simulink model "ECGdenoising_systemgenerator"  (R2018a)
settings: Solver=VariableStepAuto  StartTime=0.0  StopTime=10800  RelTol=1e-3
libraries: xbsIndex_r4 x811, dspsrcs4 x1
(part 3 of 3)

== system ECGdenoising_systemgenerator/DWT block Reference Signal generation/Low Pass Reconstruction 4 ==
  In3 : Inport
  AddSub{14..20} (7 alike) : xbsIndex_r4/AddSub  mode=Addition  use_carryin=off  use_carryout=off  en=off  latency=0  precision=User Defined  arith_type="Signed  (2's comp)"  n_bits=16  bin_pt=14  quantization=Truncate  overflow=Saturate  use_behavioral_HDL=off  hw_selection=Fabric  pipelined=off  dbl_ovrd=off  block_type=addsub
  Constant16 : xbsIndex_r4/Constant  const=0.6308807679  gui_display_data_type=Fixed-point  arith_type=Signed (2's comp)  n_bits=16  bin_pt=14  preci_type=Single  exp_width=8  frac_width=24  explicit_period=on  period=64  equ=P=C  opselect=C  inp2=PCIN>>17  opr=+  inp1=P  carry=CIN  dbl_ovrd=off  block_type=constant
  Constant17 : xbsIndex_r4/Constant  const=-0.0279837694  gui_display_data_type=Fixed-point  arith_type=Signed (2's comp)  n_bits=16  bin_pt=14  preci_type=Single  exp_width=8  frac_width=24  explicit_period=on  period=64  equ=P=C  opselect=C  inp2=PCIN>>17  opr=+  inp1=P  carry=CIN  dbl_ovrd=off  block_type=constant
  Constant18 : xbsIndex_r4/Constant  const=-0.1870348117  gui_display_data_type=Fixed-point  arith_type=Signed (2's comp)  n_bits=16  bin_pt=14  preci_type=Single  exp_width=8  frac_width=24  explicit_period=on  period=64  equ=P=C  opselect=C  inp2=PCIN>>17  opr=+  inp1=P  carry=CIN  dbl_ovrd=off  block_type=constant
  Constant19 : xbsIndex_r4/Constant  const=0.0308413818  gui_display_data_type=Fixed-point  arith_type=Signed (2's comp)  n_bits=16  bin_pt=14  preci_type=Single  exp_width=8  frac_width=24  explicit_period=on  period=64  equ=P=C  opselect=C  inp2=PCIN>>17  opr=+  inp1=P  carry=CIN  dbl_ovrd=off  block_type=constant
  Constant20 : xbsIndex_r4/Constant  const=0.0328830117  gui_display_data_type=Fixed-point  arith_type=Signed (2's comp)  n_bits=16  bin_pt=14  preci_type=Single  exp_width=8  frac_width=24  explicit_period=on  period=64  equ=P=C  opselect=C  inp2=PCIN>>17  opr=+  inp1=P  carry=CIN  dbl_ovrd=off  block_type=constant
  Constant21 : xbsIndex_r4/Constant  const=-0.0105974018  gui_display_data_type=Fixed-point  arith_type=Signed (2's comp)  n_bits=16  bin_pt=14  preci_type=Single  exp_width=8  frac_width=24  explicit_period=on  period=64  equ=P=C  opselect=C  inp2=PCIN>>17  opr=+  inp1=P  carry=CIN  dbl_ovrd=off  block_type=constant
  Constant22 : xbsIndex_r4/Constant  const=0.2303778133  gui_display_data_type=Fixed-point  arith_type=Signed (2's comp)  n_bits=16  bin_pt=14  preci_type=Single  exp_width=8  frac_width=24  explicit_period=on  period=64  equ=P=C  opselect=C  inp2=PCIN>>17  opr=+  inp1=P  carry=CIN  dbl_ovrd=off  block_type=constant
  Constant23 : xbsIndex_r4/Constant  const=0.7148465706  gui_display_data_type=Fixed-point  arith_type=Signed (2's comp)  n_bits=16  bin_pt=14  preci_type=Single  exp_width=8  frac_width=24  explicit_period=on  period=64  equ=P=C  opselect=C  inp2=PCIN>>17  opr=+  inp1=P  carry=CIN  dbl_ovrd=off  block_type=constant
  Delay{14..20} (7 alike) : xbsIndex_r4/Delay  rst=off  infoeditControl=Selection of Reset will increase slice count due to use of real FFs and instead of SRLs  en=off  latency=1  reg_retiming=off  dbl_ovrd=off  block_type=delay
      settings: infoedit=Hardware notes: A delay line is a chain, each link of which is an SRL16 or SRL32 followed by a flip-flop.
  Mult{1,16..22} (8 alike) : xbsIndex_r4/Mult  precision=User Defined  arith_type="Signed  (2's comp)"  n_bits=32  bin_pt=28  quantization=Truncate  overflow=Saturate  en=off  latency=0  use_behavioral_HDL=off  opt=Speed  use_embedded=on  optimum_pipeline=off  pipeline=on  dbl_ovrd=off  use_rpm=on  placement_style=Triangular  block_type=mult
  Out3 : Outport
  wires:
  In3/1 -> Mult22/2, Delay18/1
  Constant21/1 -> Mult21/1
  Mult21/1 -> AddSub17/1
  AddSub17/1 -> Out3/1
  AddSub16/1 -> AddSub17/2
  Constant22/1 -> Mult22/1
  Constant17/1 -> Mult17/1
  Delay14/1 -> Mult18/2, Delay15/1
  Constant18/1 -> Mult18/1
  Mult18/1 -> AddSub14/1
  AddSub20/1 -> AddSub14/2
  Constant19/1 -> Mult19/1
  Mult19/1 -> AddSub15/1
  Mult1/1 -> AddSub18/1
  AddSub14/1 -> AddSub15/2
  Delay16/1 -> Mult20/2, Delay17/1
  Constant20/1 -> Mult20/1
  AddSub15/1 -> AddSub16/2
  Mult20/1 -> AddSub16/1
  Constant23/1 -> Mult1/1
  Constant16/1 -> Mult16/1
  Delay17/1 -> Mult21/2
  Mult16/1 -> AddSub19/1
  Delay18/1 -> Mult1/2, Delay19/1
  Mult22/1 -> AddSub18/2
  Delay19/1 -> Mult16/2, Delay20/1
  AddSub18/1 -> AddSub19/2
  Delay20/1 -> Mult17/2, Delay14/1
  Delay15/1 -> Mult19/2, Delay16/1
  Mult17/1 -> AddSub20/1
  AddSub19/1 -> AddSub20/2

== system ECGdenoising_systemgenerator/DWT block Reference Signal generation/Low Pass Reconstruction 5 ==
  In3 : Inport
  AddSub{14..20} (7 alike) : xbsIndex_r4/AddSub  mode=Addition  use_carryin=off  use_carryout=off  en=off  latency=0  precision=User Defined  arith_type="Signed  (2's comp)"  n_bits=16  bin_pt=14  quantization=Truncate  overflow=Saturate  use_behavioral_HDL=off  hw_selection=Fabric  pipelined=off  dbl_ovrd=off  block_type=addsub
  Constant16 : xbsIndex_r4/Constant  const=0.6308807679  gui_display_data_type=Fixed-point  arith_type=Signed (2's comp)  n_bits=16  bin_pt=14  preci_type=Single  exp_width=8  frac_width=24  explicit_period=on  period=8  equ=P=C  opselect=C  inp2=PCIN>>17  opr=+  inp1=P  carry=CIN  dbl_ovrd=off  block_type=constant
  Constant17 : xbsIndex_r4/Constant  const=-0.0279837694  gui_display_data_type=Fixed-point  arith_type=Signed (2's comp)  n_bits=16  bin_pt=14  preci_type=Single  exp_width=8  frac_width=24  explicit_period=on  period=8  equ=P=C  opselect=C  inp2=PCIN>>17  opr=+  inp1=P  carry=CIN  dbl_ovrd=off  block_type=constant
  Constant18 : xbsIndex_r4/Constant  const=-0.1870348117  gui_display_data_type=Fixed-point  arith_type=Signed (2's comp)  n_bits=16  bin_pt=14  preci_type=Single  exp_width=8  frac_width=24  explicit_period=on  period=8  equ=P=C  opselect=C  inp2=PCIN>>17  opr=+  inp1=P  carry=CIN  dbl_ovrd=off  block_type=constant
  Constant19 : xbsIndex_r4/Constant  const=0.0308413818  gui_display_data_type=Fixed-point  arith_type=Signed (2's comp)  n_bits=16  bin_pt=14  preci_type=Single  exp_width=8  frac_width=24  explicit_period=on  period=8  equ=P=C  opselect=C  inp2=PCIN>>17  opr=+  inp1=P  carry=CIN  dbl_ovrd=off  block_type=constant
  Constant20 : xbsIndex_r4/Constant  const=0.0328830117  gui_display_data_type=Fixed-point  arith_type=Signed (2's comp)  n_bits=16  bin_pt=14  preci_type=Single  exp_width=8  frac_width=24  explicit_period=on  period=8  equ=P=C  opselect=C  inp2=PCIN>>17  opr=+  inp1=P  carry=CIN  dbl_ovrd=off  block_type=constant
  Constant21 : xbsIndex_r4/Constant  const=-0.0105974018  gui_display_data_type=Fixed-point  arith_type=Signed (2's comp)  n_bits=16  bin_pt=14  preci_type=Single  exp_width=8  frac_width=24  explicit_period=on  period=8  equ=P=C  opselect=C  inp2=PCIN>>17  opr=+  inp1=P  carry=CIN  dbl_ovrd=off  block_type=constant
  Constant22 : xbsIndex_r4/Constant  const=0.2303778133  gui_display_data_type=Fixed-point  arith_type=Signed (2's comp)  n_bits=16  bin_pt=14  preci_type=Single  exp_width=8  frac_width=24  explicit_period=on  period=8  equ=P=C  opselect=C  inp2=PCIN>>17  opr=+  inp1=P  carry=CIN  dbl_ovrd=off  block_type=constant
  Constant23 : xbsIndex_r4/Constant  const=0.7148465706  gui_display_data_type=Fixed-point  arith_type=Signed (2's comp)  n_bits=16  bin_pt=14  preci_type=Single  exp_width=8  frac_width=24  explicit_period=on  period=8  equ=P=C  opselect=C  inp2=PCIN>>17  opr=+  inp1=P  carry=CIN  dbl_ovrd=off  block_type=constant
  Delay{14..20} (7 alike) : xbsIndex_r4/Delay  rst=off  infoeditControl=Selection of Reset will increase slice count due to use of real FFs and instead of SRLs  en=off  latency=1  reg_retiming=off  dbl_ovrd=off  block_type=delay
      settings: infoedit=Hardware notes: A delay line is a chain, each link of which is an SRL16 or SRL32 followed by a flip-flop.
  Mult{1,16..22} (8 alike) : xbsIndex_r4/Mult  precision=User Defined  arith_type="Signed  (2's comp)"  n_bits=32  bin_pt=28  quantization=Truncate  overflow=Saturate  en=off  latency=0  use_behavioral_HDL=off  opt=Speed  use_embedded=on  optimum_pipeline=off  pipeline=on  dbl_ovrd=off  use_rpm=on  placement_style=Triangular  block_type=mult
  Out3 : Outport
  wires:
  In3/1 -> Mult22/2, Delay18/1
  Constant21/1 -> Mult21/1
  Mult21/1 -> AddSub17/1
  AddSub17/1 -> Out3/1
  AddSub16/1 -> AddSub17/2
  Constant22/1 -> Mult22/1
  Constant17/1 -> Mult17/1
  Delay14/1 -> Mult18/2, Delay15/1
  Constant18/1 -> Mult18/1
  Mult18/1 -> AddSub14/1
  AddSub20/1 -> AddSub14/2
  Constant19/1 -> Mult19/1
  Mult19/1 -> AddSub15/1
  Mult1/1 -> AddSub18/1
  AddSub14/1 -> AddSub15/2
  Delay16/1 -> Mult20/2, Delay17/1
  Constant20/1 -> Mult20/1
  AddSub15/1 -> AddSub16/2
  Mult20/1 -> AddSub16/1
  Constant23/1 -> Mult1/1
  Constant16/1 -> Mult16/1
  Delay17/1 -> Mult21/2
  Mult16/1 -> AddSub19/1
  Delay18/1 -> Mult1/2, Delay19/1
  Mult22/1 -> AddSub18/2
  Delay19/1 -> Mult16/2, Delay20/1
  AddSub18/1 -> AddSub19/2
  Delay20/1 -> Mult17/2, Delay14/1
  Delay15/1 -> Mult19/2, Delay16/1
  Mult17/1 -> AddSub20/1
  AddSub19/1 -> AddSub20/2

== system ECGdenoising_systemgenerator/DWT block Reference Signal generation/Low Pass Reconstruction 6 ==
  In3 : Inport
  AddSub{14..20} (7 alike) : xbsIndex_r4/AddSub  mode=Addition  use_carryin=off  use_carryout=off  en=off  latency=0  precision=User Defined  arith_type="Signed  (2's comp)"  n_bits=16  bin_pt=14  quantization=Truncate  overflow=Saturate  use_behavioral_HDL=off  hw_selection=Fabric  pipelined=off  dbl_ovrd=off  block_type=addsub
  Constant16 : xbsIndex_r4/Constant  const=0.6308807679  gui_display_data_type=Fixed-point  arith_type=Signed (2's comp)  n_bits=16  bin_pt=14  preci_type=Single  exp_width=8  frac_width=24  explicit_period=on  period=16  equ=P=C  opselect=C  inp2=PCIN>>17  opr=+  inp1=P  carry=CIN  dbl_ovrd=off  block_type=constant
  Constant17 : xbsIndex_r4/Constant  const=-0.0279837694  gui_display_data_type=Fixed-point  arith_type=Signed (2's comp)  n_bits=16  bin_pt=14  preci_type=Single  exp_width=8  frac_width=24  explicit_period=on  period=16  equ=P=C  opselect=C  inp2=PCIN>>17  opr=+  inp1=P  carry=CIN  dbl_ovrd=off  block_type=constant
  Constant18 : xbsIndex_r4/Constant  const=-0.1870348117  gui_display_data_type=Fixed-point  arith_type=Signed (2's comp)  n_bits=16  bin_pt=14  preci_type=Single  exp_width=8  frac_width=24  explicit_period=on  period=16  equ=P=C  opselect=C  inp2=PCIN>>17  opr=+  inp1=P  carry=CIN  dbl_ovrd=off  block_type=constant
  Constant19 : xbsIndex_r4/Constant  const=0.0308413818  gui_display_data_type=Fixed-point  arith_type=Signed (2's comp)  n_bits=16  bin_pt=14  preci_type=Single  exp_width=8  frac_width=24  explicit_period=on  period=16  equ=P=C  opselect=C  inp2=PCIN>>17  opr=+  inp1=P  carry=CIN  dbl_ovrd=off  block_type=constant
  Constant20 : xbsIndex_r4/Constant  const=0.0328830117  gui_display_data_type=Fixed-point  arith_type=Signed (2's comp)  n_bits=16  bin_pt=14  preci_type=Single  exp_width=8  frac_width=24  explicit_period=on  period=16  equ=P=C  opselect=C  inp2=PCIN>>17  opr=+  inp1=P  carry=CIN  dbl_ovrd=off  block_type=constant
  Constant21 : xbsIndex_r4/Constant  const=-0.0105974018  gui_display_data_type=Fixed-point  arith_type=Signed (2's comp)  n_bits=16  bin_pt=14  preci_type=Single  exp_width=8  frac_width=24  explicit_period=on  period=16  equ=P=C  opselect=C  inp2=PCIN>>17  opr=+  inp1=P  carry=CIN  dbl_ovrd=off  block_type=constant
  Constant22 : xbsIndex_r4/Constant  const=0.2303778133  gui_display_data_type=Fixed-point  arith_type=Signed (2's comp)  n_bits=16  bin_pt=14  preci_type=Single  exp_width=8  frac_width=24  explicit_period=on  period=16  equ=P=C  opselect=C  inp2=PCIN>>17  opr=+  inp1=P  carry=CIN  dbl_ovrd=off  block_type=constant
  Constant23 : xbsIndex_r4/Constant  const=0.7148465706  gui_display_data_type=Fixed-point  arith_type=Signed (2's comp)  n_bits=16  bin_pt=14  preci_type=Single  exp_width=8  frac_width=24  explicit_period=on  period=16  equ=P=C  opselect=C  inp2=PCIN>>17  opr=+  inp1=P  carry=CIN  dbl_ovrd=off  block_type=constant
  Delay{14..20} (7 alike) : xbsIndex_r4/Delay  rst=off  infoeditControl=Selection of Reset will increase slice count due to use of real FFs and instead of SRLs  en=off  latency=1  reg_retiming=off  dbl_ovrd=off  block_type=delay
      settings: infoedit=Hardware notes: A delay line is a chain, each link of which is an SRL16 or SRL32 followed by a flip-flop.
  Mult{1,16..22} (8 alike) : xbsIndex_r4/Mult  precision=User Defined  arith_type="Signed  (2's comp)"  n_bits=32  bin_pt=28  quantization=Truncate  overflow=Saturate  en=off  latency=0  use_behavioral_HDL=off  opt=Speed  use_embedded=on  optimum_pipeline=off  pipeline=on  dbl_ovrd=off  use_rpm=on  placement_style=Triangular  block_type=mult
  Out3 : Outport
  wires:
  In3/1 -> Mult22/2, Delay18/1
  Constant21/1 -> Mult21/1
  Mult21/1 -> AddSub17/1
  AddSub17/1 -> Out3/1
  AddSub16/1 -> AddSub17/2
  Constant22/1 -> Mult22/1
  Constant17/1 -> Mult17/1
  Delay14/1 -> Mult18/2, Delay15/1
  Constant18/1 -> Mult18/1
  Mult18/1 -> AddSub14/1
  AddSub20/1 -> AddSub14/2
  Constant19/1 -> Mult19/1
  Mult19/1 -> AddSub15/1
  Mult1/1 -> AddSub18/1
  AddSub14/1 -> AddSub15/2
  Delay16/1 -> Mult20/2, Delay17/1
  Constant20/1 -> Mult20/1
  AddSub15/1 -> AddSub16/2
  Mult20/1 -> AddSub16/1
  Constant23/1 -> Mult1/1
  Constant16/1 -> Mult16/1
  Delay17/1 -> Mult21/2
  Mult16/1 -> AddSub19/1
  Delay18/1 -> Mult1/2, Delay19/1
  Mult22/1 -> AddSub18/2
  Delay19/1 -> Mult16/2, Delay20/1
  AddSub18/1 -> AddSub19/2
  Delay20/1 -> Mult17/2, Delay14/1
  Delay15/1 -> Mult19/2, Delay16/1
  Mult17/1 -> AddSub20/1
  AddSub19/1 -> AddSub20/2

== system ECGdenoising_systemgenerator/DWT block Reference Signal generation/Low Pass Reconstruction 8 ==
  In3 : Inport
  AddSub{14..20} (7 alike) : xbsIndex_r4/AddSub  mode=Addition  use_carryin=off  use_carryout=off  en=off  latency=0  precision=User Defined  arith_type="Signed  (2's comp)"  n_bits=16  bin_pt=14  quantization=Truncate  overflow=Saturate  use_behavioral_HDL=off  hw_selection=Fabric  pipelined=off  dbl_ovrd=off  block_type=addsub
  Constant16 : xbsIndex_r4/Constant  const=0.6308807679  gui_display_data_type=Fixed-point  arith_type=Signed (2's comp)  n_bits=16  bin_pt=14  preci_type=Single  exp_width=8  frac_width=24  explicit_period=on  period=4  equ=P=C  opselect=C  inp2=PCIN>>17  opr=+  inp1=P  carry=CIN  dbl_ovrd=off  block_type=constant
  Constant17 : xbsIndex_r4/Constant  const=-0.0279837694  gui_display_data_type=Fixed-point  arith_type=Signed (2's comp)  n_bits=16  bin_pt=14  preci_type=Single  exp_width=8  frac_width=24  explicit_period=on  period=4  equ=P=C  opselect=C  inp2=PCIN>>17  opr=+  inp1=P  carry=CIN  dbl_ovrd=off  block_type=constant
  Constant18 : xbsIndex_r4/Constant  const=-0.1870348117  gui_display_data_type=Fixed-point  arith_type=Signed (2's comp)  n_bits=16  bin_pt=14  preci_type=Single  exp_width=8  frac_width=24  explicit_period=on  period=4  equ=P=C  opselect=C  inp2=PCIN>>17  opr=+  inp1=P  carry=CIN  dbl_ovrd=off  block_type=constant
  Constant19 : xbsIndex_r4/Constant  const=0.0308413818  gui_display_data_type=Fixed-point  arith_type=Signed (2's comp)  n_bits=16  bin_pt=14  preci_type=Single  exp_width=8  frac_width=24  explicit_period=on  period=4  equ=P=C  opselect=C  inp2=PCIN>>17  opr=+  inp1=P  carry=CIN  dbl_ovrd=off  block_type=constant
  Constant20 : xbsIndex_r4/Constant  const=0.0328830117  gui_display_data_type=Fixed-point  arith_type=Signed (2's comp)  n_bits=16  bin_pt=14  preci_type=Single  exp_width=8  frac_width=24  explicit_period=on  period=4  equ=P=C  opselect=C  inp2=PCIN>>17  opr=+  inp1=P  carry=CIN  dbl_ovrd=off  block_type=constant
  Constant21 : xbsIndex_r4/Constant  const=-0.0105974018  gui_display_data_type=Fixed-point  arith_type=Signed (2's comp)  n_bits=16  bin_pt=14  preci_type=Single  exp_width=8  frac_width=24  explicit_period=on  period=4  equ=P=C  opselect=C  inp2=PCIN>>17  opr=+  inp1=P  carry=CIN  dbl_ovrd=off  block_type=constant
  Constant22 : xbsIndex_r4/Constant  const=0.2303778133  gui_display_data_type=Fixed-point  arith_type=Signed (2's comp)  n_bits=16  bin_pt=14  preci_type=Single  exp_width=8  frac_width=24  explicit_period=on  period=4  equ=P=C  opselect=C  inp2=PCIN>>17  opr=+  inp1=P  carry=CIN  dbl_ovrd=off  block_type=constant
  Constant23 : xbsIndex_r4/Constant  const=0.7148465706  gui_display_data_type=Fixed-point  arith_type=Signed (2's comp)  n_bits=16  bin_pt=14  preci_type=Single  exp_width=8  frac_width=24  explicit_period=on  period=4  equ=P=C  opselect=C  inp2=PCIN>>17  opr=+  inp1=P  carry=CIN  dbl_ovrd=off  block_type=constant
  Delay{14..20} (7 alike) : xbsIndex_r4/Delay  rst=off  infoeditControl=Selection of Reset will increase slice count due to use of real FFs and instead of SRLs  en=off  latency=1  reg_retiming=off  dbl_ovrd=off  block_type=delay
      settings: infoedit=Hardware notes: A delay line is a chain, each link of which is an SRL16 or SRL32 followed by a flip-flop.
  Mult{1,16..22} (8 alike) : xbsIndex_r4/Mult  precision=User Defined  arith_type="Signed  (2's comp)"  n_bits=32  bin_pt=28  quantization=Truncate  overflow=Saturate  en=off  latency=0  use_behavioral_HDL=off  opt=Speed  use_embedded=on  optimum_pipeline=off  pipeline=on  dbl_ovrd=off  use_rpm=on  placement_style=Triangular  block_type=mult
  Out3 : Outport
  wires:
  In3/1 -> Mult22/2, Delay18/1
  Constant21/1 -> Mult21/1
  Mult21/1 -> AddSub17/1
  AddSub17/1 -> Out3/1
  AddSub16/1 -> AddSub17/2
  Constant22/1 -> Mult22/1
  Constant17/1 -> Mult17/1
  Delay14/1 -> Mult18/2, Delay15/1
  Constant18/1 -> Mult18/1
  Mult18/1 -> AddSub14/1
  AddSub20/1 -> AddSub14/2
  Constant19/1 -> Mult19/1
  Mult19/1 -> AddSub15/1
  Mult1/1 -> AddSub18/1
  AddSub14/1 -> AddSub15/2
  Delay16/1 -> Mult20/2, Delay17/1
  Constant20/1 -> Mult20/1
  AddSub15/1 -> AddSub16/2
  Mult20/1 -> AddSub16/1
  Constant23/1 -> Mult1/1
  Constant16/1 -> Mult16/1
  Delay17/1 -> Mult21/2
  Mult16/1 -> AddSub19/1
  Delay18/1 -> Mult1/2, Delay19/1
  Mult22/1 -> AddSub18/2
  Delay19/1 -> Mult16/2, Delay20/1
  AddSub18/1 -> AddSub19/2
  Delay20/1 -> Mult17/2, Delay14/1
  Delay15/1 -> Mult19/2, Delay16/1
  Mult17/1 -> AddSub20/1
  AddSub19/1 -> AddSub20/2

== system ECGdenoising_systemgenerator/DWT block Reference Signal generation/Low Pass Reconstruction 9 ==
  In3 : Inport
  AddSub{14..20} (7 alike) : xbsIndex_r4/AddSub  mode=Addition  use_carryin=off  use_carryout=off  en=off  latency=0  precision=User Defined  arith_type="Signed  (2's comp)"  n_bits=16  bin_pt=14  quantization=Truncate  overflow=Saturate  use_behavioral_HDL=off  hw_selection=Fabric  pipelined=off  dbl_ovrd=off  block_type=addsub
  Constant16 : xbsIndex_r4/Constant  const=0.6308807679  gui_display_data_type=Fixed-point  arith_type=Signed (2's comp)  n_bits=16  bin_pt=14  preci_type=Single  exp_width=8  frac_width=24  explicit_period=on  period=1  equ=P=C  opselect=C  inp2=PCIN>>17  opr=+  inp1=P  carry=CIN  dbl_ovrd=off  block_type=constant
  Constant17 : xbsIndex_r4/Constant  const=-0.0279837694  gui_display_data_type=Fixed-point  arith_type=Signed (2's comp)  n_bits=16  bin_pt=14  preci_type=Single  exp_width=8  frac_width=24  explicit_period=on  period=1  equ=P=C  opselect=C  inp2=PCIN>>17  opr=+  inp1=P  carry=CIN  dbl_ovrd=off  block_type=constant
  Constant18 : xbsIndex_r4/Constant  const=-0.1870348117  gui_display_data_type=Fixed-point  arith_type=Signed (2's comp)  n_bits=16  bin_pt=14  preci_type=Single  exp_width=8  frac_width=24  explicit_period=on  period=1  equ=P=C  opselect=C  inp2=PCIN>>17  opr=+  inp1=P  carry=CIN  dbl_ovrd=off  block_type=constant
  Constant19 : xbsIndex_r4/Constant  const=0.0308413818  gui_display_data_type=Fixed-point  arith_type=Signed (2's comp)  n_bits=16  bin_pt=14  preci_type=Single  exp_width=8  frac_width=24  explicit_period=on  period=1  equ=P=C  opselect=C  inp2=PCIN>>17  opr=+  inp1=P  carry=CIN  dbl_ovrd=off  block_type=constant
  Constant20 : xbsIndex_r4/Constant  const=0.0328830117  gui_display_data_type=Fixed-point  arith_type=Signed (2's comp)  n_bits=16  bin_pt=14  preci_type=Single  exp_width=8  frac_width=24  explicit_period=on  period=1  equ=P=C  opselect=C  inp2=PCIN>>17  opr=+  inp1=P  carry=CIN  dbl_ovrd=off  block_type=constant
  Constant21 : xbsIndex_r4/Constant  const=-0.0105974018  gui_display_data_type=Fixed-point  arith_type=Signed (2's comp)  n_bits=16  bin_pt=14  preci_type=Single  exp_width=8  frac_width=24  explicit_period=on  period=1  equ=P=C  opselect=C  inp2=PCIN>>17  opr=+  inp1=P  carry=CIN  dbl_ovrd=off  block_type=constant
  Constant22 : xbsIndex_r4/Constant  const=0.2303778133  gui_display_data_type=Fixed-point  arith_type=Signed (2's comp)  n_bits=16  bin_pt=14  preci_type=Single  exp_width=8  frac_width=24  explicit_period=on  period=1  equ=P=C  opselect=C  inp2=PCIN>>17  opr=+  inp1=P  carry=CIN  dbl_ovrd=off  block_type=constant
  Constant23 : xbsIndex_r4/Constant  const=0.7148465706  gui_display_data_type=Fixed-point  arith_type=Signed (2's comp)  n_bits=16  bin_pt=14  preci_type=Single  exp_width=8  frac_width=24  explicit_period=on  period=1  equ=P=C  opselect=C  inp2=PCIN>>17  opr=+  inp1=P  carry=CIN  dbl_ovrd=off  block_type=constant
  Delay{14..20} (7 alike) : xbsIndex_r4/Delay  rst=off  infoeditControl=Selection of Reset will increase slice count due to use of real FFs and instead of SRLs  en=off  latency=1  reg_retiming=off  dbl_ovrd=off  block_type=delay
      settings: infoedit=Hardware notes: A delay line is a chain, each link of which is an SRL16 or SRL32 followed by a flip-flop.
  Mult{1,16..22} (8 alike) : xbsIndex_r4/Mult  precision=User Defined  arith_type="Signed  (2's comp)"  n_bits=32  bin_pt=28  quantization=Truncate  overflow=Saturate  en=off  latency=0  use_behavioral_HDL=off  opt=Speed  use_embedded=on  optimum_pipeline=off  pipeline=on  dbl_ovrd=off  use_rpm=on  placement_style=Triangular  block_type=mult
  Out3 : Outport
  wires:
  In3/1 -> Mult22/2, Delay18/1
  Constant21/1 -> Mult21/1
  Mult21/1 -> AddSub17/1
  AddSub17/1 -> Out3/1
  AddSub16/1 -> AddSub17/2
  Constant22/1 -> Mult22/1
  Constant17/1 -> Mult17/1
  Delay14/1 -> Mult18/2, Delay15/1
  Constant18/1 -> Mult18/1
  Mult18/1 -> AddSub14/1
  AddSub20/1 -> AddSub14/2
  Constant19/1 -> Mult19/1
  Mult19/1 -> AddSub15/1
  Mult1/1 -> AddSub18/1
  AddSub14/1 -> AddSub15/2
  Delay16/1 -> Mult20/2, Delay17/1
  Constant20/1 -> Mult20/1
  AddSub15/1 -> AddSub16/2
  Mult20/1 -> AddSub16/1
  Constant23/1 -> Mult1/1
  Constant16/1 -> Mult16/1
  Delay17/1 -> Mult21/2
  Mult16/1 -> AddSub19/1
  Delay18/1 -> Mult1/2, Delay19/1
  Mult22/1 -> AddSub18/2
  Delay19/1 -> Mult16/2, Delay20/1
  AddSub18/1 -> AddSub19/2
  Delay20/1 -> Mult17/2, Delay14/1
  Delay15/1 -> Mult19/2, Delay16/1
  Mult17/1 -> AddSub20/1
  AddSub19/1 -> AddSub20/2

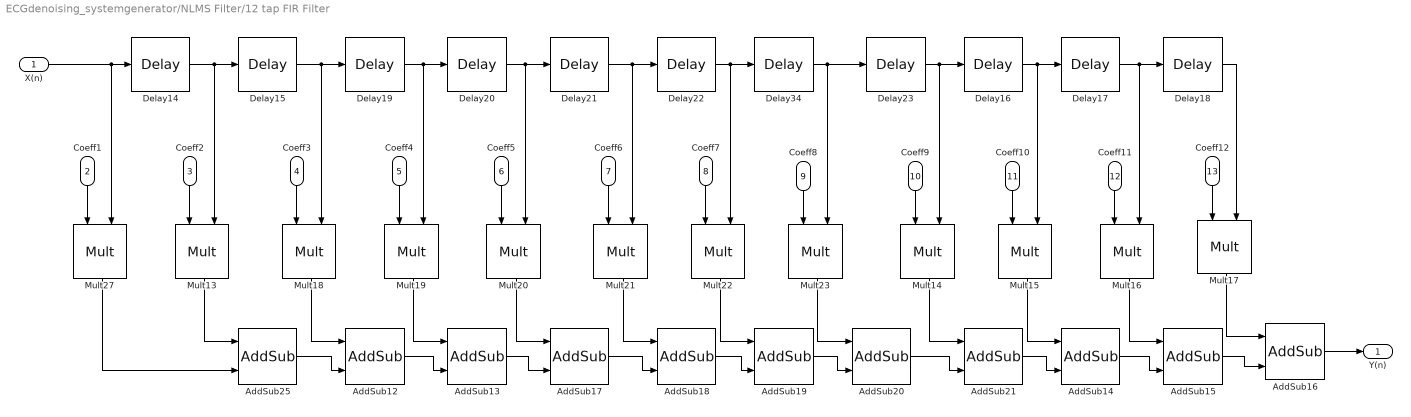
== system ECGdenoising_systemgenerator/NLMS Filter/12 tap FIR Filter ==
  "X(n) " : Inport  SampleTime=1
  Coeff1 : Inport  Port=2  SampleTime=1
  Coeff2 : Inport  Port=3  SampleTime=1
  Coeff3 : Inport  Port=4  SampleTime=1
  Coeff4 : Inport  Port=5  SampleTime=1
  Coeff5 : Inport  Port=6  SampleTime=1
  Coeff6 : Inport  Port=7  SampleTime=1
  Coeff7 : Inport  Port=8  SampleTime=1
  Coeff8 : Inport  Port=9  SampleTime=1
  Coeff9 : Inport  Port=10  SampleTime=1
  Coeff10 : Inport  Port=11  SampleTime=1
  Coeff11 : Inport  Port=12  SampleTime=1
  Coeff12 : Inport  Port=13  SampleTime=1
  AddSub{12..21,25} (11 alike) : xbsIndex_r4/AddSub  mode=Addition  use_carryin=off  use_carryout=off  en=off  latency=0  precision=User Defined  arith_type="Signed  (2's comp)"  n_bits=16  bin_pt=14  quantization=Truncate  overflow=Saturate  use_behavioral_HDL=off  hw_selection=Fabric  pipelined=off  dbl_ovrd=off  block_type=addsub
  Delay{14..23,34} (11 alike) : xbsIndex_r4/Delay  rst=off  infoeditControl=Selection of Reset will increase slice count due to use of real FFs and instead of SRLs  en=off  latency=1  reg_retiming=off  dbl_ovrd=off  block_type=delay
      Delay22 settings: infoedit=Hardware notes: A delay line is a chain, each link of which is an SRL16 or SRL32 followed by a flip-flop.
  Mult{13..23,27} (12 alike) : xbsIndex_r4/Mult  precision=User Defined  arith_type="Signed  (2's comp)"  n_bits=32  bin_pt=28  quantization=Truncate  overflow=Saturate  en=off  latency=0  use_behavioral_HDL=off  opt=Speed  use_embedded=on  optimum_pipeline=off  pipeline=on  dbl_ovrd=off  use_rpm=on  placement_style=Triangular  block_type=mult
  Y(n) : Outport  SampleTime=1
  wires:
  Delay17/1 -> Mult16/2, Delay18/1
  Mult23/1 -> AddSub20/1
  Coeff3/1 -> Mult18/1
  AddSub17/1 -> AddSub18/2
  Coeff7/1 -> Mult22/1
  Mult18/1 -> AddSub12/1
  Delay14/1 -> Mult13/2, Delay15/1
  AddSub19/1 -> AddSub20/2
  Coeff2/1 -> Mult13/1
  AddSub12/1 -> AddSub13/2
  Mult13/1 -> AddSub25/1
  Coeff10/1 -> Mult15/1
  Delay20/1 -> Mult20/2, Delay21/1
  AddSub25/1 -> AddSub12/2
  Mult27/1 -> AddSub25/2
  Delay15/1 -> Mult18/2, Delay19/1
  Mult20/1 -> AddSub17/1
  Coeff5/1 -> Mult20/1
  Delay22/1 -> Mult22/2, Delay34/1
  AddSub15/1 -> AddSub16/2
  Mult22/1 -> AddSub19/1
  Delay34/1 -> Delay23/1, Mult23/2
  AddSub16/1 -> Y(n)/1
  Coeff1/1 -> Mult27/1
  Coeff6/1 -> Mult21/1
  Delay19/1 -> Mult19/2, Delay20/1
  "X(n) "/1 -> Mult27/2, Delay14/1
  Delay16/1 -> Mult15/2, Delay17/1
  AddSub13/1 -> AddSub17/2
  Coeff12/1 -> Mult17/1
  Delay18/1 -> Mult17/2
  Mult21/1 -> AddSub18/1
  Mult17/1 -> AddSub16/1
  Delay21/1 -> Mult21/2, Delay22/1
  AddSub14/1 -> AddSub15/2
  Mult19/1 -> AddSub13/1
  Coeff9/1 -> Mult14/1
  Coeff11/1 -> Mult16/1
  Coeff8/1 -> Mult23/1
  Delay23/1 -> Mult14/2, Delay16/1
  AddSub20/1 -> AddSub21/2
  Coeff4/1 -> Mult19/1
  Mult14/1 -> AddSub21/1
  Mult16/1 -> AddSub15/1
  AddSub18/1 -> AddSub19/2
  AddSub21/1 -> AddSub14/2
  Mult15/1 -> AddSub14/1

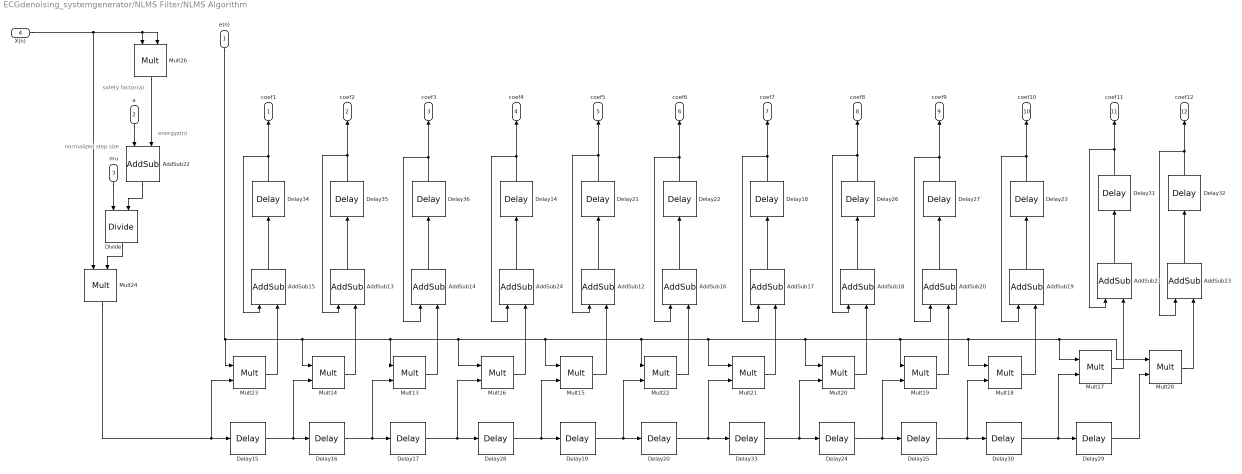
== system ECGdenoising_systemgenerator/NLMS Filter/NLMS Algorithm ==
  note: energyx(n)
  note: normalized step size
  note: safety factor(a)
  e(n) : Inport  SampleTime=1
  a : Inport  Port=2  SampleTime=1
  mu : Inport  Port=3  SampleTime=1
  X(n) : Inport  Port=4  SampleTime=1
  AddSub{12..24} (13 alike) : xbsIndex_r4/AddSub  mode=Addition  use_carryin=off  use_carryout=off  en=off  latency=0  precision=User Defined  arith_type="Signed  (2's comp)"  n_bits=16  bin_pt=14  quantization=Truncate  overflow=Saturate  use_behavioral_HDL=off  hw_selection=Fabric  pipelined=off  dbl_ovrd=off  block_type=addsub
  Delay{14..36} (23 alike) : xbsIndex_r4/Delay  rst=off  infoeditControl=Selection of Reset will increase slice count due to use of real FFs and instead of SRLs  en=off  latency=1  reg_retiming=off  dbl_ovrd=off  block_type=delay
      settings: infoedit=Hardware notes: A delay line is a chain, each link of which is an SRL16 or SRL32 followed by a flip-flop.
  Divide : xbsIndex_r4/Divide  flow_control=NonBlocking  axi_optimize_goal=Resources  algorithm_type=Radix2  infoedit1=Specify output fraction-width for Fixed-point division.  fractional_width=14  infoedit2=Specify latency for Floating-point division.  latency=1  rate=1  has_a_tlast=off  has_a_tuser=off  has_b_tlast=off  has_b_tuser=off  en=off  has_result_tready=off  result_tlast_behv=Pass_A_TLAST  has_underflow=off  has_overflow=off  has_invalid_op=off  has_divide_by_zero=off  fpo_op_type=mergeddivide  block_type=divide
      settings: infoedit=Blocking: Wait for data on all inputs, allow back-pressure.<br>NonBlocking: operate every cycle in which all inputs are valid, no back-pressure.
  Mult{13..24,26,28} (14 alike) : xbsIndex_r4/Mult  precision=User Defined  arith_type="Signed  (2's comp)"  n_bits=32  bin_pt=28  quantization=Truncate  overflow=Saturate  en=off  latency=0  use_behavioral_HDL=off  opt=Speed  use_embedded=on  optimum_pipeline=off  pipeline=on  dbl_ovrd=off  use_rpm=on  placement_style=Triangular  block_type=mult
  coef1 : Outport  SampleTime=1
  coef2 : Outport  Port=2  SampleTime=1
  coef3 : Outport  Port=3  SampleTime=1
  coef4 : Outport  Port=4  SampleTime=1
  coef5 : Outport  Port=5  SampleTime=1
  coef6 : Outport  Port=6  SampleTime=1
  coef7 : Outport  Port=7  SampleTime=1
  coef8 : Outport  Port=8  SampleTime=1
  coef9 : Outport  Port=9  SampleTime=1
  coef10 : Outport  Port=10  SampleTime=1
  coef11 : Outport  Port=11  SampleTime=1
  coef12 : Outport  Port=12  SampleTime=1
  wires:
  AddSub24/1 -> Delay14/1
  e(n)/1 -> Mult14/1, Mult13/1, Mult16/1, Mult15/1, Mult22/1, Mult21/1, Mult20/1, Mult19/1, Mult18/1, Mult17/1, Mult28/1, Mult23/1
  Delay21/1 -> coef5/1, AddSub12/1
  Mult26/1 -> AddSub22/2
  Delay22/1 -> coef6/1, AddSub16/1
  AddSub21/1 -> Delay31/1
  Delay25/1 -> Mult18/2, Delay30/1
  Delay16/1 -> Mult13/2, Delay17/1
  AddSub19/1 -> Delay23/1
  Delay17/1 -> Mult16/2, Delay28/1
  Mult16/1 -> AddSub24/2
  Delay32/1 -> coef12/1, AddSub23/1
  Mult21/1 -> AddSub17/2
  Delay31/1 -> coef11/1, AddSub21/1
  Delay24/1 -> Mult19/2, Delay25/1
  Delay34/1 -> coef1/1, AddSub15/1
  Delay14/1 -> coef4/1, AddSub24/1
  Delay19/1 -> Mult22/2, Delay20/1
  Delay30/1 -> Mult17/2, Delay29/1
  Delay35/1 -> coef2/1, AddSub13/1
  Delay15/1 -> Mult14/2, Delay16/1
  Delay20/1 -> Mult21/2, Delay33/1
  Delay36/1 -> coef3/1, AddSub14/1
  AddSub15/1 -> Delay34/1
  Mult18/1 -> AddSub19/2
  Mult28/1 -> AddSub23/2
  AddSub20/1 -> Delay27/1
  Mult14/1 -> AddSub13/2
  AddSub23/1 -> Delay32/1
  AddSub18/1 -> Delay26/1
  X(n)/1 -> Mult26/2, Mult26/1, Mult24/1
  AddSub16/1 -> Delay22/1
  Mult13/1 -> AddSub14/2
  a/1 -> AddSub22/1
  Delay28/1 -> Mult15/2, Delay19/1
  Mult23/1 -> AddSub15/2
  AddSub14/1 -> Delay36/1
  Mult24/1 -> Mult23/2, Delay15/1
  Mult22/1 -> AddSub16/2
  Delay27/1 -> coef9/1, AddSub20/1
  mu/1 -> Divide/1
  AddSub22/1 -> Divide/2
  Mult17/1 -> AddSub21/2
  Mult19/1 -> AddSub20/2
  Delay33/1 -> Mult20/2, Delay24/1
  Delay26/1 -> coef8/1, AddSub18/1
  Mult20/1 -> AddSub18/2
  Delay23/1 -> coef10/1, AddSub19/1
  Delay29/1 -> Mult28/2
  Divide/1 -> Mult24/2
  Mult15/1 -> AddSub12/2
  Delay18/1 -> coef7/1, AddSub17/1
  AddSub17/1 -> Delay18/1
  AddSub13/1 -> Delay35/1
  AddSub12/1 -> Delay21/1
